simulink model "without_treatment"  (R2021b)
settings: Solver=VariableStepAuto  StartTime=0.0  StopTime=90000  RelTol=1e-3
settings Model: Creator=Rasoul  LastModifiedBy=Rasoul
settings SolverCC: AlgebraicLoopSolver=TrustRegion
settings DebuggingCC: ArithmeticOperatorsInVariantConditions=warning
settings SFSimCC: CustomCodeUndefinedFunction=UseInterfaceOnly

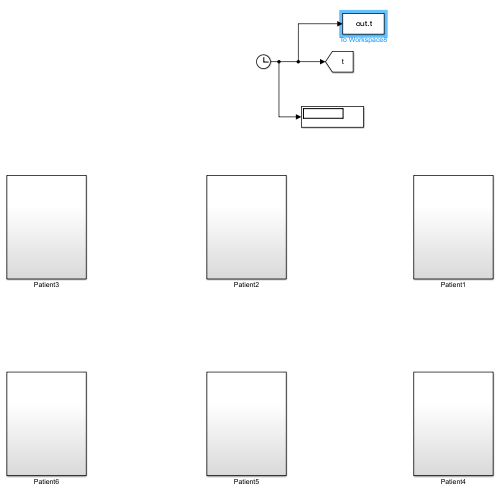
[thumbnail: Simulink's stored preview of the top-level diagram]
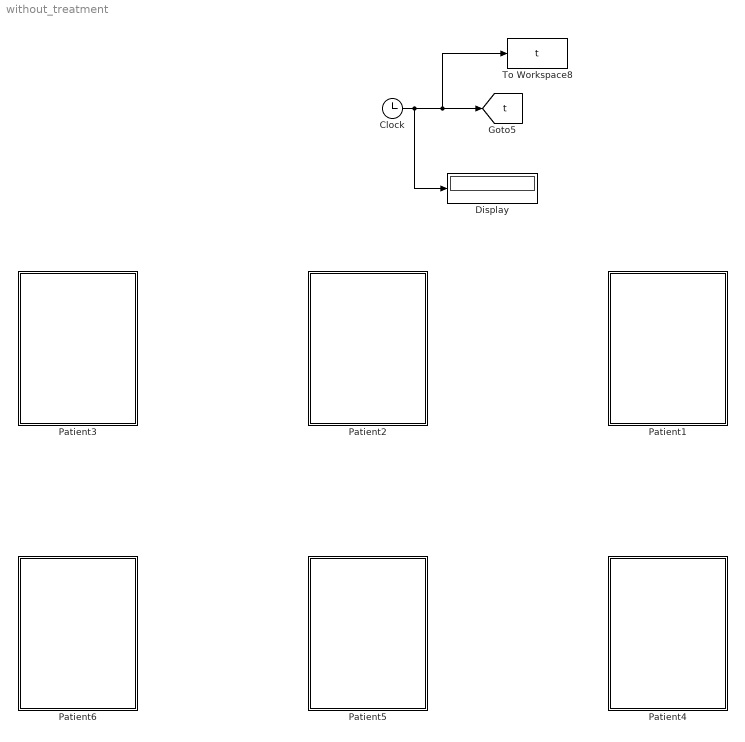
== system without_treatment ==
  Clock : Clock
  Display : Display
  Patient1 : Subsystem
  Patient2 : Subsystem
  Patient3 : Subsystem
  Patient4 : Subsystem
  Patient5 : Subsystem
  Patient6 : Subsystem
  To Workspace8 : ToWorkspace  VariableName=t  SampleTime=10
      settings: Save2DSignal=2-D array (concatenate along first dimension)
  tag scope: t=global
  wires:
  Clock/1 -> Display/1, To Workspace8/1, [t]

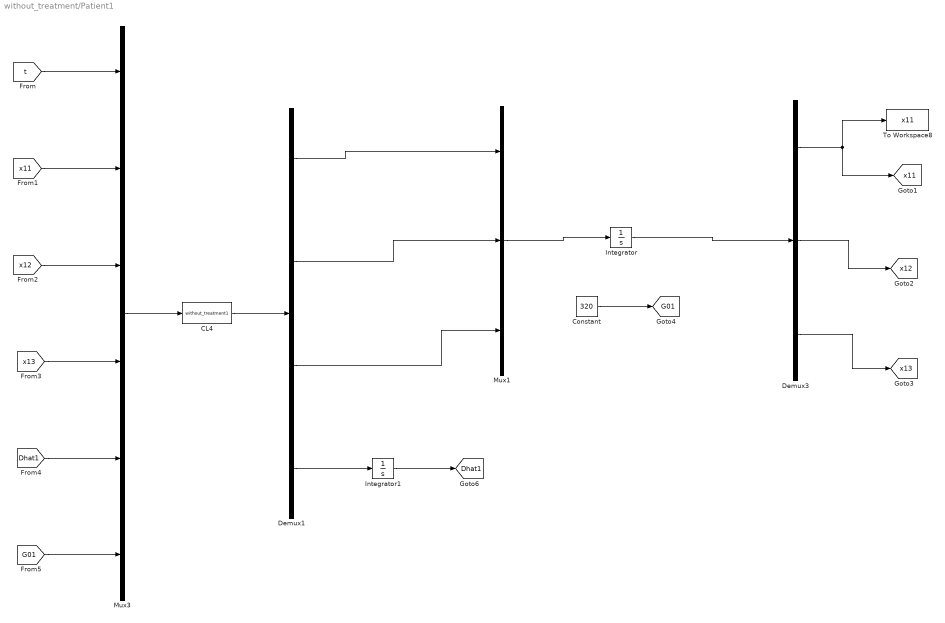
== system without_treatment/Patient1 ==
  CL4 : MATLABFcn  MATLABFcn=without_treatment1  OutputDimensions=4
  Constant : Constant  Value=320
  Demux1 : Demux
  Demux3 : Demux  Outputs=3
  Integrator : Integrator  InitialCondition=[320;0;100]
  Integrator1 : Integrator
  Mux1 : Mux  Inputs=3
  Mux3 : Mux  Inputs=6
  To Workspace8 : ToWorkspace  VariableName=x11  SampleTime=10
      settings: Save2DSignal=2-D array (concatenate along first dimension)
  tag scope: Dhat1=global, G01=global, x11=global, x12=global, x13=global
  wires:
  [x11] -> Mux3/2
  Demux3/1 -> To Workspace8/1, [x11]
  CL4/1 -> Demux1/1
  [x12] -> Mux3/3
  Demux1/4 -> Integrator1/1
  Mux1/1 -> Integrator/1
  [Dhat1] -> Mux3/5
  Demux1/2 -> Mux1/2
  [x13] -> Mux3/4
  Mux3/1 -> CL4/1
  Demux3/2 -> [x12]
  Demux1/1 -> Mux1/1
  Integrator/1 -> Demux3/1
  Demux1/3 -> Mux1/3
  Integrator1/1 -> [Dhat1]
  [t] -> Mux3/1
  Demux3/3 -> [x13]
  [G01] -> Mux3/6
  Constant/1 -> [G01]

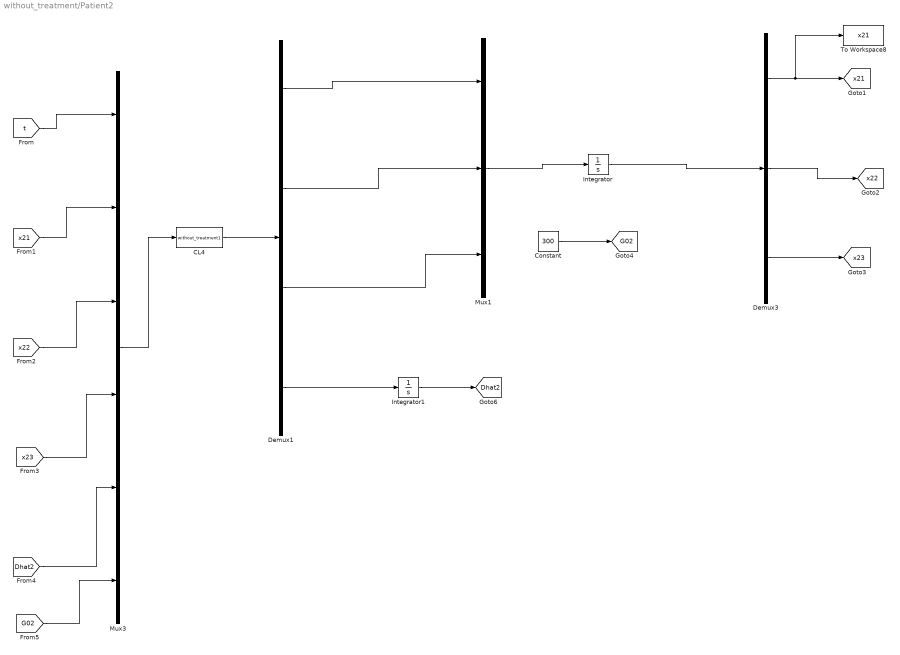
== system without_treatment/Patient2 ==
  CL4 : MATLABFcn  MATLABFcn=without_treatment1  OutputDimensions=4
  Constant : Constant  Value=300
  Demux1 : Demux
  Demux3 : Demux  Outputs=3
  Integrator : Integrator  InitialCondition=[300;0;100]
  Integrator1 : Integrator
  Mux1 : Mux  Inputs=3
  Mux3 : Mux  Inputs=6
  To Workspace8 : ToWorkspace  VariableName=x21  SampleTime=10
      settings: Save2DSignal=2-D array (concatenate along first dimension)
  tag scope: Dhat2=global, G02=global, x21=global, x22=global, x23=global
  wires:
  Demux1/4 -> Integrator1/1
  CL4/1 -> Demux1/1
  [t] -> Mux3/1
  [x21] -> Mux3/2
  Demux1/3 -> Mux1/3
  Integrator/1 -> Demux3/1
  Demux3/3 -> [x23]
  Demux3/2 -> [x22]
  [x23] -> Mux3/4
  Demux1/1 -> Mux1/1
  Mux1/1 -> Integrator/1
  Mux3/1 -> CL4/1
  Demux1/2 -> Mux1/2
  [Dhat2] -> Mux3/5
  [x22] -> Mux3/3
  Integrator1/1 -> [Dhat2]
  Constant/1 -> [G02]
  [G02] -> Mux3/6
  Demux3/1 -> To Workspace8/1, [x21]

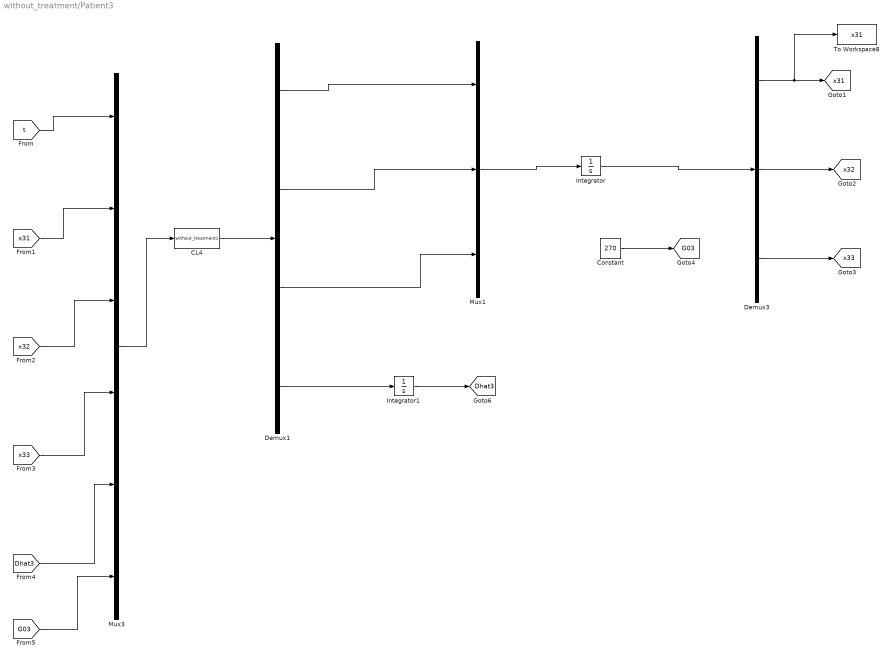
== system without_treatment/Patient3 ==
  CL4 : MATLABFcn  MATLABFcn=without_treatment1  OutputDimensions=4
  Constant : Constant  Value=270
  Demux1 : Demux
  Demux3 : Demux  Outputs=3
  Integrator : Integrator  InitialCondition=[270;0;100]
  Integrator1 : Integrator
  Mux1 : Mux  Inputs=3
  Mux3 : Mux  Inputs=6
  To Workspace8 : ToWorkspace  VariableName=x31  SampleTime=10
      settings: Save2DSignal=2-D array (concatenate along first dimension)
  tag scope: Dhat3=global, G03=global, x31=global, x32=global, x33=global
  wires:
  [Dhat3] -> Mux3/5
  Demux1/2 -> Mux1/2
  Mux3/1 -> CL4/1
  Mux1/1 -> Integrator/1
  [x33] -> Mux3/4
  Demux1/1 -> Mux1/1
  Demux3/2 -> [x32]
  Integrator/1 -> Demux3/1
  Demux3/3 -> [x33]
  Integrator1/1 -> [Dhat3]
  [x31] -> Mux3/2
  Demux1/3 -> Mux1/3
  Demux1/4 -> Integrator1/1
  [x32] -> Mux3/3
  [t] -> Mux3/1
  CL4/1 -> Demux1/1
  Constant/1 -> [G03]
  [G03] -> Mux3/6
  Demux3/1 -> To Workspace8/1, [x31]

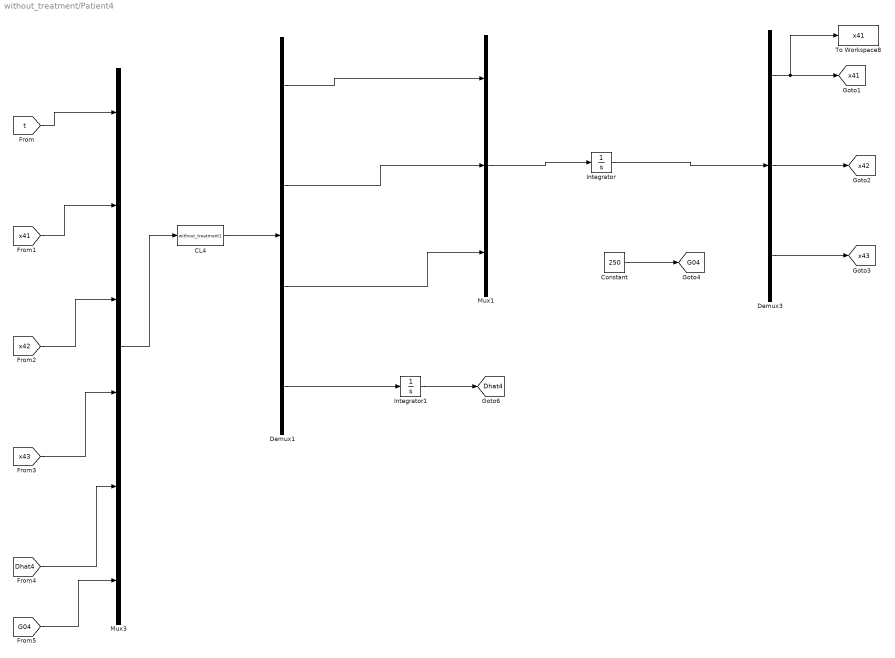
== system without_treatment/Patient4 ==
  CL4 : MATLABFcn  MATLABFcn=without_treatment1  OutputDimensions=4
  Constant : Constant  Value=250
  Demux1 : Demux
  Demux3 : Demux  Outputs=3
  Integrator : Integrator  InitialCondition=[250;0;100]
  Integrator1 : Integrator
  Mux1 : Mux  Inputs=3
  Mux3 : Mux  Inputs=6
  To Workspace8 : ToWorkspace  VariableName=x41  SampleTime=10
      settings: Save2DSignal=2-D array (concatenate along first dimension)
  tag scope: Dhat4=global, G04=global, x41=global, x42=global, x43=global
  wires:
  [t] -> Mux3/1
  CL4/1 -> Demux1/1
  Demux1/4 -> Integrator1/1
  Demux1/3 -> Mux1/3
  Integrator1/1 -> [Dhat4]
  Demux3/3 -> [x43]
  Integrator/1 -> Demux3/1
  [x41] -> Mux3/2
  Mux1/1 -> Integrator/1
  Demux3/2 -> [x42]
  [x43] -> Mux3/4
  [x42] -> Mux3/3
  Mux3/1 -> CL4/1
  Demux1/1 -> Mux1/1
  Demux1/2 -> Mux1/2
  [Dhat4] -> Mux3/5
  Constant/1 -> [G04]
  [G04] -> Mux3/6
  Demux3/1 -> To Workspace8/1, [x41]

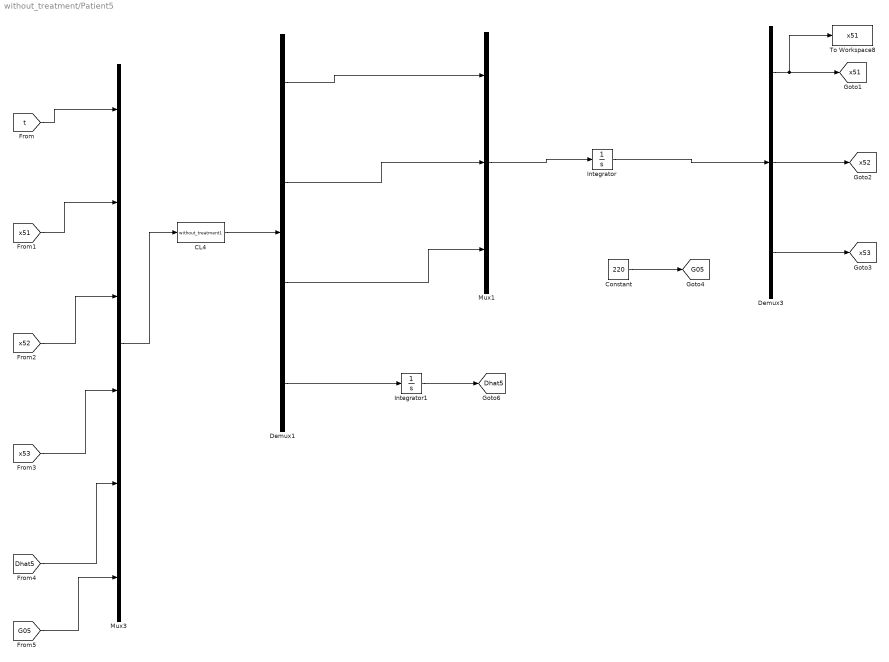
== system without_treatment/Patient5 ==
  CL4 : MATLABFcn  MATLABFcn=without_treatment1  OutputDimensions=4
  Constant : Constant  Value=220
  Demux1 : Demux
  Demux3 : Demux  Outputs=3
  Integrator : Integrator  InitialCondition=[220;0;100]
  Integrator1 : Integrator
  Mux1 : Mux  Inputs=3
  Mux3 : Mux  Inputs=6
  To Workspace8 : ToWorkspace  VariableName=x51  SampleTime=10
      settings: Save2DSignal=2-D array (concatenate along first dimension)
  tag scope: Dhat5=global, G05=global, x51=global, x52=global, x53=global
  wires:
  [t] -> Mux3/1
  CL4/1 -> Demux1/1
  Demux1/4 -> Integrator1/1
  Demux1/3 -> Mux1/3
  Integrator1/1 -> [Dhat5]
  Demux3/3 -> [x53]
  Integrator/1 -> Demux3/1
  [x51] -> Mux3/2
  Mux1/1 -> Integrator/1
  Demux3/2 -> [x52]
  [x53] -> Mux3/4
  [x52] -> Mux3/3
  Mux3/1 -> CL4/1
  Demux1/1 -> Mux1/1
  Demux1/2 -> Mux1/2
  [Dhat5] -> Mux3/5
  Constant/1 -> [G05]
  [G05] -> Mux3/6
  Demux3/1 -> To Workspace8/1, [x51]

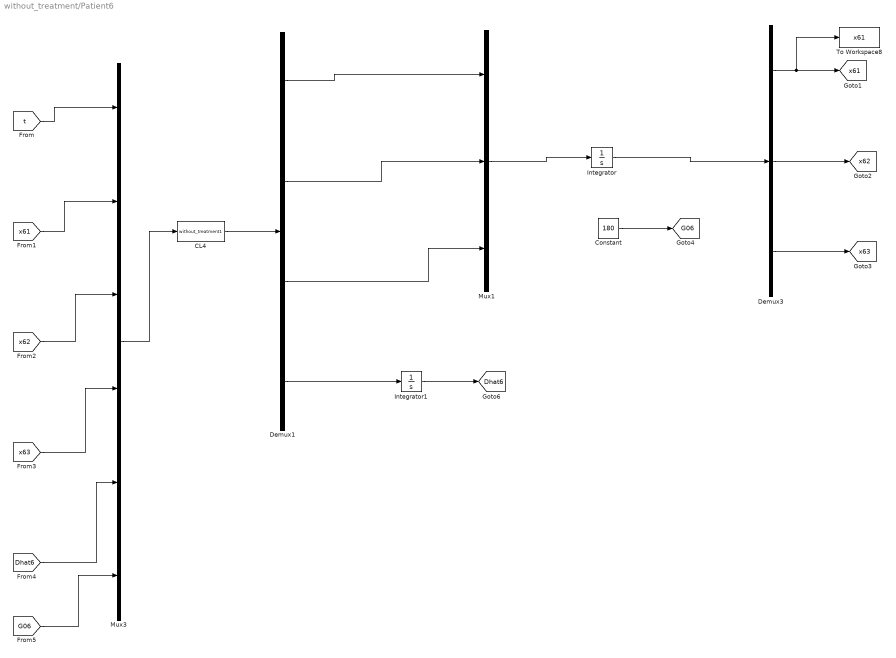
== system without_treatment/Patient6 ==
  CL4 : MATLABFcn  MATLABFcn=without_treatment1  OutputDimensions=4
  Constant : Constant  Value=180
  Demux1 : Demux
  Demux3 : Demux  Outputs=3
  Integrator : Integrator  InitialCondition=[180;0;100]
  Integrator1 : Integrator
  Mux1 : Mux  Inputs=3
  Mux3 : Mux  Inputs=6
  To Workspace8 : ToWorkspace  VariableName=x61  SampleTime=10
      settings: Save2DSignal=2-D array (concatenate along first dimension)
  tag scope: Dhat6=global, G06=global, x61=global, x62=global, x63=global
  wires:
  [t] -> Mux3/1
  CL4/1 -> Demux1/1
  Demux1/4 -> Integrator1/1
  Demux1/3 -> Mux1/3
  Integrator1/1 -> [Dhat6]
  Demux3/3 -> [x63]
  Integrator/1 -> Demux3/1
  [x61] -> Mux3/2
  Mux1/1 -> Integrator/1
  Demux3/2 -> [x62]
  [x63] -> Mux3/4
  [x62] -> Mux3/3
  Mux3/1 -> CL4/1
  Demux1/1 -> Mux1/1
  Demux1/2 -> Mux1/2
  [Dhat6] -> Mux3/5
  Constant/1 -> [G06]
  [G06] -> Mux3/6
  Demux3/1 -> To Workspace8/1, [x61]
